simulink model "ADLK"  (R2022a)
settings: Solver=FixedStepDiscrete  StartTime=0.0  StopTime=10.0  FixedStep=0.01  RelTol=1e-3
libraries: simulink x4, DoorRatSts x4, ADLKDriver x2
settings Model: Creator=DELL  LastModifiedBy=DELL
settings DataIOCC: SaveFormat=StructureWithTime
settings OptimizationCC: DefaultParameterBehavior=Inlined  EnhancedBackFolding=on  PassReuseOutputArgsAs=Individual arguments  ZeroExternalMemoryAtStartup=off  ZeroInternalMemoryAtStartup=off  OptimizeBlockOrder=speed  DifferentSizesBufferReuse=on  OptimizationCustomize=off  EfficientTunableParamExpr=on
settings DebuggingCC: ParameterTunabilityLossMsg=error
settings ModelReferenceCC: ModelReferenceNumInstancesAllowed=Single
settings SFSimCC: MATLABDynamicMemAlloc=off
settings RTWCC: Description=AUTOSAR  SystemTargetFile=autosar.tlc  GenCodeOnly=on  TemplateMakefile=ert_default_tmf
settings CodeAppCC: ForceParamTrailComments=on  IgnoreCustomStorageClasses=off  OperatorAnnotations=on  SimulinkDataObjDesc=on  SFDataObjDesc=on  InsertBlockDesc=on
settings STFCustomTargetCC: TargetLangStandard=C99 (ISO)  MultiwordLength=256  ParMdlRefBuildCompliant=on  CompOptLevelCompliant=on  IncludeMdlTerminateFcn=off  CombineOutputUpdateFcns=on  SuppressErrorStatus=on  ERTCustomFileBanners=on  SupportNonFinite=off  SupportComplex=off  SupportContinuousTime=off  SupportNonInlinedSFcns=off  RemoveResetFunc=on  MATLABClassNameForMDSCustomization=Simulink.SoftwareTarget.ERTCustomization  AutosarCompliant=on  GRTInterface=off  UseToolchainInfoCompliant=on  LookupTableObjectStructAxisOrder=2,1,3,4,...  LUTObjectStructOrderEvenSpacing=Size,Table,Breakpoints  SystemTargetFile=autosar.tlc
settings ERTTargetCC: TargetLangStandard=C99 (ISO)  ConcurrentExecutionCompliant=off  IncludeMdlTerminateFcn=off  SuppressErrorStatus=on  SupportNonFinite=off  SupportComplex=off  ModelStepFunctionPrototypeControlCompliant=off  CPPClassGenCompliant=off  AutosarCompliant=on  LookupTableObjectStructAxisOrder=2,1,3,4,...  LUTObjectStructOrderEvenSpacing=Size,Table,Breakpoints  InlinedParameterPlacement=NonHierarchical  ERTCustomFileTemplate=example_file_process.tlc

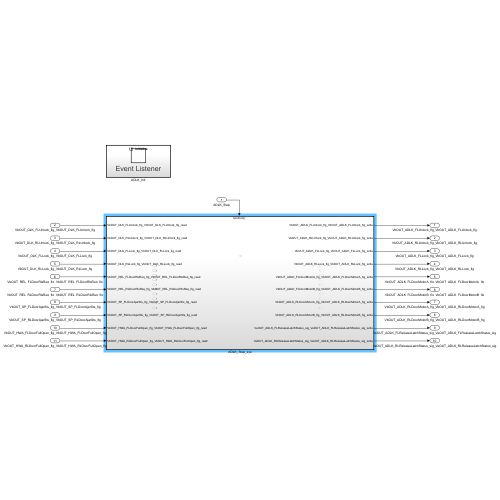
[thumbnail: Simulink's stored preview of the top-level diagram]
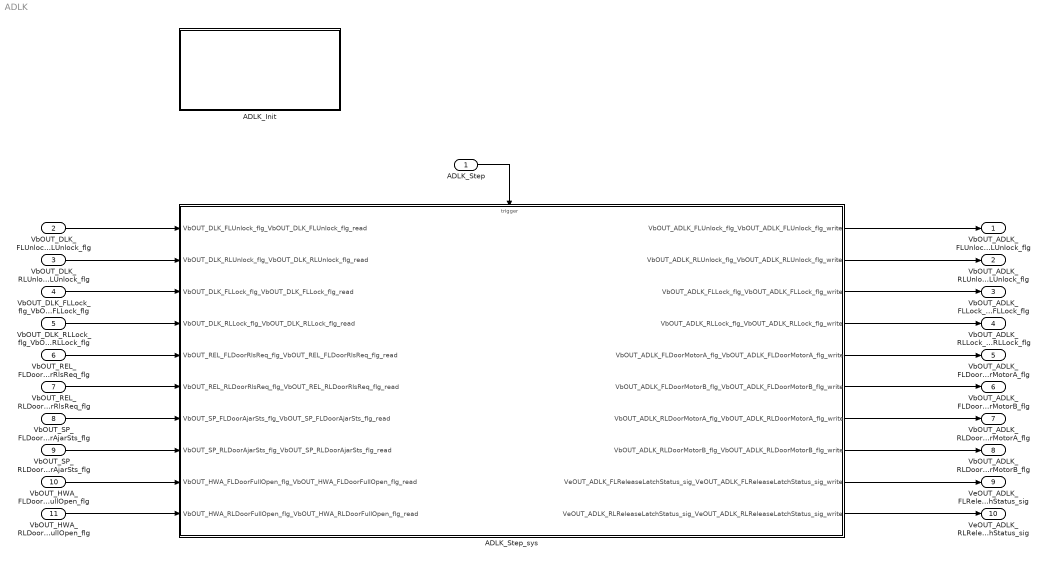
== system ADLK ==
  ADLK_Step : Inport  SampleTime=0.01  OutputFunctionCall=on
  VbOUT_DLK_FLUnlock_flg_VbOUT_DLK_FLUnlock_flg : Inport  Port=2  OutDataTypeStr=Boolean  PortDimensions=1
  VbOUT_DLK_RLUnlock_flg_VbOUT_DLK_RLUnlock_flg : Inport  Port=3  OutDataTypeStr=Boolean  PortDimensions=1
  VbOUT_DLK_FLLock_flg_VbOUT_DLK_FLLock_flg : Inport  Port=4  OutDataTypeStr=Boolean  PortDimensions=1
  VbOUT_DLK_RLLock_flg_VbOUT_DLK_RLLock_flg : Inport  Port=5  OutDataTypeStr=Boolean  PortDimensions=1
  VbOUT_REL_FLDoorRlsReq_flg_VbOUT_REL_FLDoorRlsReq_flg : Inport  Port=6  OutDataTypeStr=Boolean  PortDimensions=1
  VbOUT_REL_RLDoorRlsReq_flg_VbOUT_REL_RLDoorRlsReq_flg : Inport  Port=7  OutDataTypeStr=Boolean  PortDimensions=1
  VbOUT_SP_FLDoorAjarSts_flg_VbOUT_SP_FLDoorAjarSts_flg : Inport  Port=8  OutDataTypeStr=Boolean  PortDimensions=1
  VbOUT_SP_RLDoorAjarSts_flg_VbOUT_SP_RLDoorAjarSts_flg : Inport  Port=9  OutDataTypeStr=Boolean  PortDimensions=1
  VbOUT_HWA_FLDoorFullOpen_flg_VbOUT_HWA_FLDoorFullOpen_flg : Inport  Port=10  OutDataTypeStr=Boolean  PortDimensions=1
  VbOUT_HWA_RLDoorFullOpen_flg_VbOUT_HWA_RLDoorFullOpen_flg : Inport  Port=11  OutDataTypeStr=Boolean  PortDimensions=1
  ADLK_Init : Subsystem
  ADLK_Step_sys : Subsystem
  VbOUT_ADLK_FLUnlock_flg_VbOUT_ADLK_FLUnlock_flg : Outport  OutDataTypeStr=Boolean  PortDimensions=1
  VbOUT_ADLK_RLUnlock_flg_VbOUT_ADLK_RLUnlock_flg : Outport  Port=2  OutDataTypeStr=Boolean  PortDimensions=1
  VbOUT_ADLK_FLLock_flg_VbOUT_ADLK_FLLock_flg : Outport  Port=3  OutDataTypeStr=Boolean  PortDimensions=1
  VbOUT_ADLK_RLLock_flg_VbOUT_ADLK_RLLock_flg : Outport  Port=4  OutDataTypeStr=Boolean  PortDimensions=1
  VbOUT_ADLK_FLDoorMotorA_flg_VbOUT_ADLK_FLDoorMotorA_flg : Outport  Port=5  OutDataTypeStr=Boolean  PortDimensions=1
  VbOUT_ADLK_FLDoorMotorB_flg_VbOUT_ADLK_FLDoorMotorB_flg : Outport  Port=6  OutDataTypeStr=Boolean  PortDimensions=1
  VbOUT_ADLK_RLDoorMotorA_flg_VbOUT_ADLK_RLDoorMotorA_flg : Outport  Port=7  OutDataTypeStr=Boolean  PortDimensions=1
  VbOUT_ADLK_RLDoorMotorB_flg_VbOUT_ADLK_RLDoorMotorB_flg : Outport  Port=8  OutDataTypeStr=Boolean  PortDimensions=1
  VeOUT_ADLK_FLReleaseLatchStatus_sig_VeOUT_ADLK_FLReleaseLatchStatus_sig : Outport  Port=9  OutDataTypeStr=UInt8  PortDimensions=1
  VeOUT_ADLK_RLReleaseLatchStatus_sig_VeOUT_ADLK_RLReleaseLatchStatus_sig : Outport  Port=10  OutDataTypeStr=UInt8  PortDimensions=1
  wires:
  VbOUT_DLK_FLUnlock_flg_VbOUT_DLK_FLUnlock_flg/1 -> ADLK_Step_sys/1(VbOUT_DLK_FLUnlock_flg_VbOUT_DLK_FLUnlock_flg_read)
  VbOUT_DLK_RLUnlock_flg_VbOUT_DLK_RLUnlock_flg/1 -> ADLK_Step_sys/2(VbOUT_DLK_RLUnlock_flg_VbOUT_DLK_RLUnlock_flg_read)
  VbOUT_DLK_FLLock_flg_VbOUT_DLK_FLLock_flg/1 -> ADLK_Step_sys/3(VbOUT_DLK_FLLock_flg_VbOUT_DLK_FLLock_flg_read)
  VbOUT_DLK_RLLock_flg_VbOUT_DLK_RLLock_flg/1 -> ADLK_Step_sys/4(VbOUT_DLK_RLLock_flg_VbOUT_DLK_RLLock_flg_read)
  VbOUT_REL_FLDoorRlsReq_flg_VbOUT_REL_FLDoorRlsReq_flg/1 -> ADLK_Step_sys/5(VbOUT_REL_FLDoorRlsReq_flg_VbOUT_REL_FLDoorRlsReq_flg_read)
  VbOUT_REL_RLDoorRlsReq_flg_VbOUT_REL_RLDoorRlsReq_flg/1 -> ADLK_Step_sys/6(VbOUT_REL_RLDoorRlsReq_flg_VbOUT_REL_RLDoorRlsReq_flg_read)
  VbOUT_SP_FLDoorAjarSts_flg_VbOUT_SP_FLDoorAjarSts_flg/1 -> ADLK_Step_sys/7(VbOUT_SP_FLDoorAjarSts_flg_VbOUT_SP_FLDoorAjarSts_flg_read)
  VbOUT_SP_RLDoorAjarSts_flg_VbOUT_SP_RLDoorAjarSts_flg/1 -> ADLK_Step_sys/8(VbOUT_SP_RLDoorAjarSts_flg_VbOUT_SP_RLDoorAjarSts_flg_read)
  VbOUT_HWA_FLDoorFullOpen_flg_VbOUT_HWA_FLDoorFullOpen_flg/1 -> ADLK_Step_sys/9(VbOUT_HWA_FLDoorFullOpen_flg_VbOUT_HWA_FLDoorFullOpen_flg_read)
  VbOUT_HWA_RLDoorFullOpen_flg_VbOUT_HWA_RLDoorFullOpen_flg/1 -> ADLK_Step_sys/10(VbOUT_HWA_RLDoorFullOpen_flg_VbOUT_HWA_RLDoorFullOpen_flg_read)
  ADLK_Step_sys/1(VbOUT_ADLK_FLUnlock_flg_VbOUT_ADLK_FLUnlock_flg_write) -> VbOUT_ADLK_FLUnlock_flg_VbOUT_ADLK_FLUnlock_flg/1
  ADLK_Step_sys/2(VbOUT_ADLK_RLUnlock_flg_VbOUT_ADLK_RLUnlock_flg_write) -> VbOUT_ADLK_RLUnlock_flg_VbOUT_ADLK_RLUnlock_flg/1
  ADLK_Step_sys/3(VbOUT_ADLK_FLLock_flg_VbOUT_ADLK_FLLock_flg_write) -> VbOUT_ADLK_FLLock_flg_VbOUT_ADLK_FLLock_flg/1
  ADLK_Step_sys/4(VbOUT_ADLK_RLLock_flg_VbOUT_ADLK_RLLock_flg_write) -> VbOUT_ADLK_RLLock_flg_VbOUT_ADLK_RLLock_flg/1
  ADLK_Step_sys/5(VbOUT_ADLK_FLDoorMotorA_flg_VbOUT_ADLK_FLDoorMotorA_flg_write) -> VbOUT_ADLK_FLDoorMotorA_flg_VbOUT_ADLK_FLDoorMotorA_flg/1
  ADLK_Step_sys/6(VbOUT_ADLK_FLDoorMotorB_flg_VbOUT_ADLK_FLDoorMotorB_flg_write) -> VbOUT_ADLK_FLDoorMotorB_flg_VbOUT_ADLK_FLDoorMotorB_flg/1
  ADLK_Step_sys/7(VbOUT_ADLK_RLDoorMotorA_flg_VbOUT_ADLK_RLDoorMotorA_flg_write) -> VbOUT_ADLK_RLDoorMotorA_flg_VbOUT_ADLK_RLDoorMotorA_flg/1
  ADLK_Step_sys/8(VbOUT_ADLK_RLDoorMotorB_flg_VbOUT_ADLK_RLDoorMotorB_flg_write) -> VbOUT_ADLK_RLDoorMotorB_flg_VbOUT_ADLK_RLDoorMotorB_flg/1
  ADLK_Step_sys/9(VeOUT_ADLK_FLReleaseLatchStatus_sig_VeOUT_ADLK_FLReleaseLatchStatus_sig_write) -> VeOUT_ADLK_FLReleaseLatchStatus_sig_VeOUT_ADLK_FLReleaseLatchStatus_sig/1
  ADLK_Step_sys/10(VeOUT_ADLK_RLReleaseLatchStatus_sig_VeOUT_ADLK_RLReleaseLatchStatus_sig_write) -> VeOUT_ADLK_RLReleaseLatchStatus_sig_VeOUT_ADLK_RLReleaseLatchStatus_sig/1
  ADLK_Step/1 -> ADLK_Step_sys/Trigger

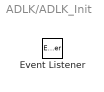
== system ADLK/ADLK_Init ==
  Event Listener : EventListener  EventName=reset

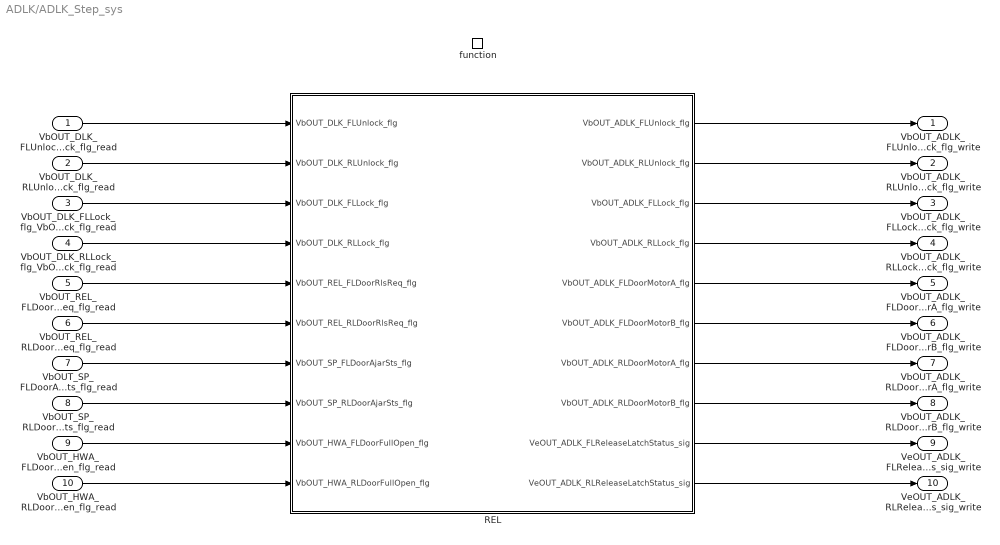
== system ADLK/ADLK_Step_sys ==
  VbOUT_DLK_FLUnlock_flg_VbOUT_DLK_FLUnlock_flg_read : Inport
  VbOUT_DLK_RLUnlock_flg_VbOUT_DLK_RLUnlock_flg_read : Inport  Port=2
  VbOUT_DLK_FLLock_flg_VbOUT_DLK_FLLock_flg_read : Inport  Port=3
  VbOUT_DLK_RLLock_flg_VbOUT_DLK_RLLock_flg_read : Inport  Port=4
  VbOUT_REL_FLDoorRlsReq_flg_VbOUT_REL_FLDoorRlsReq_flg_read : Inport  Port=5
  VbOUT_REL_RLDoorRlsReq_flg_VbOUT_REL_RLDoorRlsReq_flg_read : Inport  Port=6
  VbOUT_SP_FLDoorAjarSts_flg_VbOUT_SP_FLDoorAjarSts_flg_read : Inport  Port=7
  VbOUT_SP_RLDoorAjarSts_flg_VbOUT_SP_RLDoorAjarSts_flg_read : Inport  Port=8
  VbOUT_HWA_FLDoorFullOpen_flg_VbOUT_HWA_FLDoorFullOpen_flg_read : Inport  Port=9
  VbOUT_HWA_RLDoorFullOpen_flg_VbOUT_HWA_RLDoorFullOpen_flg_read : Inport  Port=10
  function : TriggerPort  TriggerType=function-call  VariantControl=(inherit)  SampleTimeType=periodic  SampleTime=-1
  REL : Subsystem
  VbOUT_ADLK_FLUnlock_flg_VbOUT_ADLK_FLUnlock_flg_write : Outport
      settings: EnsureOutportIsVirtual=on
  VbOUT_ADLK_RLUnlock_flg_VbOUT_ADLK_RLUnlock_flg_write : Outport  Port=2
      settings: EnsureOutportIsVirtual=on
  VbOUT_ADLK_FLLock_flg_VbOUT_ADLK_FLLock_flg_write : Outport  Port=3
      settings: EnsureOutportIsVirtual=on
  VbOUT_ADLK_RLLock_flg_VbOUT_ADLK_RLLock_flg_write : Outport  Port=4
      settings: EnsureOutportIsVirtual=on
  VbOUT_ADLK_FLDoorMotorA_flg_VbOUT_ADLK_FLDoorMotorA_flg_write : Outport  Port=5
      settings: EnsureOutportIsVirtual=on
  VbOUT_ADLK_FLDoorMotorB_flg_VbOUT_ADLK_FLDoorMotorB_flg_write : Outport  Port=6
      settings: EnsureOutportIsVirtual=on
  VbOUT_ADLK_RLDoorMotorA_flg_VbOUT_ADLK_RLDoorMotorA_flg_write : Outport  Port=7
      settings: EnsureOutportIsVirtual=on
  VbOUT_ADLK_RLDoorMotorB_flg_VbOUT_ADLK_RLDoorMotorB_flg_write : Outport  Port=8
      settings: EnsureOutportIsVirtual=on
  VeOUT_ADLK_FLReleaseLatchStatus_sig_VeOUT_ADLK_FLReleaseLatchStatus_sig_write : Outport  Port=9
      settings: EnsureOutportIsVirtual=on
  VeOUT_ADLK_RLReleaseLatchStatus_sig_VeOUT_ADLK_RLReleaseLatchStatus_sig_write : Outport  Port=10
      settings: EnsureOutportIsVirtual=on
  wires:
  REL/1(VbOUT_ADLK_FLUnlock_flg) -> VbOUT_ADLK_FLUnlock_flg_VbOUT_ADLK_FLUnlock_flg_write/1
  REL/2(VbOUT_ADLK_RLUnlock_flg) -> VbOUT_ADLK_RLUnlock_flg_VbOUT_ADLK_RLUnlock_flg_write/1
  REL/3(VbOUT_ADLK_FLLock_flg) -> VbOUT_ADLK_FLLock_flg_VbOUT_ADLK_FLLock_flg_write/1
  REL/4(VbOUT_ADLK_RLLock_flg) -> VbOUT_ADLK_RLLock_flg_VbOUT_ADLK_RLLock_flg_write/1
  REL/5(VbOUT_ADLK_FLDoorMotorA_flg) -> VbOUT_ADLK_FLDoorMotorA_flg_VbOUT_ADLK_FLDoorMotorA_flg_write/1
  REL/6(VbOUT_ADLK_FLDoorMotorB_flg) -> VbOUT_ADLK_FLDoorMotorB_flg_VbOUT_ADLK_FLDoorMotorB_flg_write/1
  REL/7(VbOUT_ADLK_RLDoorMotorA_flg) -> VbOUT_ADLK_RLDoorMotorA_flg_VbOUT_ADLK_RLDoorMotorA_flg_write/1
  REL/8(VbOUT_ADLK_RLDoorMotorB_flg) -> VbOUT_ADLK_RLDoorMotorB_flg_VbOUT_ADLK_RLDoorMotorB_flg_write/1
  REL/9(VeOUT_ADLK_FLReleaseLatchStatus_sig) -> VeOUT_ADLK_FLReleaseLatchStatus_sig_VeOUT_ADLK_FLReleaseLatchStatus_sig_write/1
  REL/10(VeOUT_ADLK_RLReleaseLatchStatus_sig) -> VeOUT_ADLK_RLReleaseLatchStatus_sig_VeOUT_ADLK_RLReleaseLatchStatus_sig_write/1
  VbOUT_DLK_FLUnlock_flg_VbOUT_DLK_FLUnlock_flg_read/1 -> REL/1(VbOUT_DLK_FLUnlock_flg)
  VbOUT_DLK_RLUnlock_flg_VbOUT_DLK_RLUnlock_flg_read/1 -> REL/2(VbOUT_DLK_RLUnlock_flg)
  VbOUT_DLK_FLLock_flg_VbOUT_DLK_FLLock_flg_read/1 -> REL/3(VbOUT_DLK_FLLock_flg)
  VbOUT_DLK_RLLock_flg_VbOUT_DLK_RLLock_flg_read/1 -> REL/4(VbOUT_DLK_RLLock_flg)
  VbOUT_REL_FLDoorRlsReq_flg_VbOUT_REL_FLDoorRlsReq_flg_read/1 -> REL/5(VbOUT_REL_FLDoorRlsReq_flg)
  VbOUT_REL_RLDoorRlsReq_flg_VbOUT_REL_RLDoorRlsReq_flg_read/1 -> REL/6(VbOUT_REL_RLDoorRlsReq_flg)
  VbOUT_SP_FLDoorAjarSts_flg_VbOUT_SP_FLDoorAjarSts_flg_read/1 -> REL/7(VbOUT_SP_FLDoorAjarSts_flg)
  VbOUT_SP_RLDoorAjarSts_flg_VbOUT_SP_RLDoorAjarSts_flg_read/1 -> REL/8(VbOUT_SP_RLDoorAjarSts_flg)
  VbOUT_HWA_FLDoorFullOpen_flg_VbOUT_HWA_FLDoorFullOpen_flg_read/1 -> REL/9(VbOUT_HWA_FLDoorFullOpen_flg)
  VbOUT_HWA_RLDoorFullOpen_flg_VbOUT_HWA_RLDoorFullOpen_flg_read/1 -> REL/10(VbOUT_HWA_RLDoorFullOpen_flg)

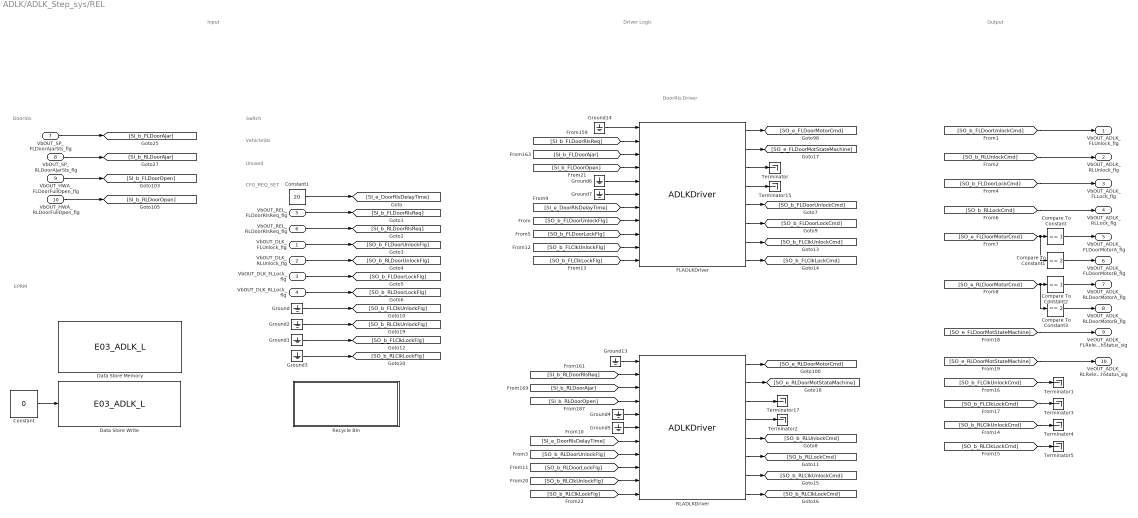
== system ADLK/ADLK_Step_sys/REL ==
  note: VehicleSts
  note: Input
  note: Output
  note: EPRM
  note: Driver Logic
  note: DoorRls Driver
  note: Switch
  note: DoorSts
  note: CFG_REQ_SET
  note: Unused
  VbOUT_DLK_FLUnlock_flg : Inport
  VbOUT_DLK_RLUnlock_flg : Inport  Port=2
  VbOUT_DLK_FLLock_flg : Inport  Port=3
  VbOUT_DLK_RLLock_flg : Inport  Port=4
  VbOUT_REL_FLDoorRlsReq_flg : Inport  Port=5
  VbOUT_REL_RLDoorRlsReq_flg : Inport  Port=6
  VbOUT_SP_FLDoorAjarSts_flg : Inport  Port=7
  VbOUT_SP_RLDoorAjarSts_flg : Inport  Port=8
  VbOUT_HWA_FLDoorFullOpen_flg : Inport  Port=9
  VbOUT_HWA_RLDoorFullOpen_flg : Inport  Port=10
  Compare To Constant : simulink/Logic and Bit Operations/Compare To Constant  relop===  const=1  OutDataTypeStr=boolean
  Compare To Constant1 : simulink/Logic and Bit Operations/Compare To Constant  relop===  const=2  OutDataTypeStr=boolean
  Compare To Constant2 : simulink/Logic and Bit Operations/Compare To Constant  relop===  const=1  OutDataTypeStr=boolean
  Compare To Constant3 : simulink/Logic and Bit Operations/Compare To Constant  relop===  const=2  OutDataTypeStr=boolean
  Constant : Constant  Value=0  OutDataTypeStr=uint8
  Constant1 : Constant  Value=20  OutDataTypeStr=uint8
  Data Store Memory : DataStoreMemory  DataStoreName=E03_ADLK_L  WriteAfterWriteMsg=warning  ShowAdditionalParam=off  OutDataTypeStr=uint8
  Data Store Write : DataStoreWrite  DataStoreName=E03_ADLK_L  IndexOptions=Index vector (dialog)  Indices=1  OutputSizes=1
  FLADLKDriver : ADLKDriver/ADLKDriver  SystemSampleTime=-1  VariantActivationTime=update diagram  Latency=0  AutoFrameSizeCalculation=off
  Ground{,1..7,13..14} (10 alike) : Ground
  RLADLKDriver : ADLKDriver/ADLKDriver  SystemSampleTime=-1  VariantActivationTime=update diagram  Latency=0  AutoFrameSizeCalculation=off
  Recycle Bin : Subsystem
  Terminator{,1..5,15,17} (8 alike) : Terminator
  VbOUT_ADLK_FLUnlock_flg : Outport
  VbOUT_ADLK_RLUnlock_flg : Outport  Port=2
  VbOUT_ADLK_FLLock_flg : Outport  Port=3
  VbOUT_ADLK_RLLock_flg : Outport  Port=4
  VbOUT_ADLK_FLDoorMotorA_flg : Outport  Port=5
  VbOUT_ADLK_FLDoorMotorB_flg : Outport  Port=6
  VbOUT_ADLK_RLDoorMotorA_flg : Outport  Port=7
  VbOUT_ADLK_RLDoorMotorB_flg : Outport  Port=8
  VeOUT_ADLK_FLReleaseLatchStatus_sig : Outport  Port=9
  VeOUT_ADLK_RLReleaseLatchStatus_sig : Outport  Port=10
  wires:
  Constant/1 -> Data Store Write/1
  [SI_b_RLDoorOpen] -> RLADLKDriver/4
  [SI_b_RLDoorAjar] -> RLADLKDriver/3
  [SI_b_RLDoorRlsReq] -> RLADLKDriver/2
  Ground13/1 -> RLADLKDriver/1
  [SI_b_FLDoorAjar] -> FLADLKDriver/3
  [SI_b_FLDoorRlsReq] -> FLADLKDriver/2
  [SI_b_FLDoorOpen] -> FLADLKDriver/4
  [SI_e_DoorRlsDelayTime] -> FLADLKDriver/7
  Ground4/1 -> RLADLKDriver/5
  Ground5/1 -> RLADLKDriver/6
  Ground6/1 -> FLADLKDriver/5
  Ground7/1 -> FLADLKDriver/6
  Ground14/1 -> FLADLKDriver/1
  Constant1/1 -> [SI_e_DoorRlsDelayTime]
  [SI_e_DoorRlsDelayTime] -> RLADLKDriver/7
  VbOUT_SP_FLDoorAjarSts_flg/1 -> [SI_b_FLDoorAjar]
  VbOUT_SP_RLDoorAjarSts_flg/1 -> [SI_b_RLDoorAjar]
  VbOUT_HWA_FLDoorFullOpen_flg/1 -> [SI_b_FLDoorOpen]
  VbOUT_HWA_RLDoorFullOpen_flg/1 -> [SI_b_RLDoorOpen]
  VbOUT_REL_FLDoorRlsReq_flg/1 -> [SI_b_FLDoorRlsReq]
  VbOUT_REL_RLDoorRlsReq_flg/1 -> [SI_b_RLDoorRlsReq]
  [SO_b_FLDoorLockFlg] -> FLADLKDriver/9
  [SO_b_FLDoorUnlockFlg] -> FLADLKDriver/8
  [SO_b_RLDoorUnlockFlg] -> RLADLKDriver/8
  [SO_b_RLDoorLockFlg] -> RLADLKDriver/9
  VbOUT_DLK_FLUnlock_flg/1 -> [SO_b_FLDoorUnlockFlg]
  VbOUT_DLK_RLUnlock_flg/1 -> [SO_b_RLDoorUnlockFlg]
  VbOUT_DLK_FLLock_flg/1 -> [SO_b_FLDoorLockFlg]
  VbOUT_DLK_RLLock_flg/1 -> [SO_b_RLDoorLockFlg]
  [SO_b_FLClkUnlockFlg] -> FLADLKDriver/10
  [SO_b_FLClkLockFlg] -> FLADLKDriver/11
  Ground/1 -> [SO_b_FLClkUnlockFlg]
  Ground1/1 -> [SO_b_FLClkLockFlg]
  [SO_b_FLDoorUnlockCmd] -> VbOUT_ADLK_FLUnlock_flg/1
  [SO_b_RLUnlockCmd] -> VbOUT_ADLK_RLUnlock_flg/1
  [SO_b_FLDoorLockCmd] -> VbOUT_ADLK_FLLock_flg/1
  [SO_b_RLLockCmd] -> VbOUT_ADLK_RLLock_flg/1
  [SO_e_FLDoorMotorCmd] -> Compare To Constant1/1, Compare To Constant/1
  Compare To Constant/1 -> VbOUT_ADLK_FLDoorMotorA_flg/1
  Compare To Constant1/1 -> VbOUT_ADLK_FLDoorMotorB_flg/1
  Compare To Constant2/1 -> VbOUT_ADLK_RLDoorMotorA_flg/1
  [SO_e_RLDoorMotorCmd] -> Compare To Constant3/1, Compare To Constant2/1
  Compare To Constant3/1 -> VbOUT_ADLK_RLDoorMotorB_flg/1
  [SO_e_FLDoorMotStateMachine] -> VeOUT_ADLK_FLReleaseLatchStatus_sig/1
  [SO_e_RLDoorMotStateMachine] -> VeOUT_ADLK_RLReleaseLatchStatus_sig/1
  [SO_b_FLClkUnlockCmd] -> Terminator1/1
  [SO_b_FLClkLockCmd] -> Terminator3/1
  [SO_b_RLClkUnlockCmd] -> Terminator4/1
  [SO_b_RLClkLockCmd] -> Terminator5/1
  FLADLKDriver/1 -> [SO_e_FLDoorMotorCmd]
  FLADLKDriver/8 -> [SO_b_FLClkLockCmd]
  FLADLKDriver/7 -> [SO_b_FLClkUnlockCmd]
  FLADLKDriver/2 -> [SO_e_FLDoorMotStateMachine]
  FLADLKDriver/6 -> [SO_b_FLDoorLockCmd]
  FLADLKDriver/5 -> [SO_b_FLDoorUnlockCmd]
  FLADLKDriver/4 -> Terminator15/1
  FLADLKDriver/3 -> Terminator/1
  RLADLKDriver/1 -> [SO_e_RLDoorMotorCmd]
  RLADLKDriver/8 -> [SO_b_RLClkLockCmd]
  RLADLKDriver/7 -> [SO_b_RLClkUnlockCmd]
  RLADLKDriver/6 -> [SO_b_RLLockCmd]
  RLADLKDriver/2 -> [SO_e_RLDoorMotStateMachine]
  RLADLKDriver/5 -> [SO_b_RLUnlockCmd]
  RLADLKDriver/4 -> Terminator2/1
  RLADLKDriver/3 -> Terminator17/1
  Ground2/1 -> [SO_b_RLClkUnlockFlg]
  Ground3/1 -> [SO_b_RLClkLockFlg]
  [SO_b_RLClkUnlockFlg] -> RLADLKDriver/10
  [SO_b_RLClkLockFlg] -> RLADLKDriver/11

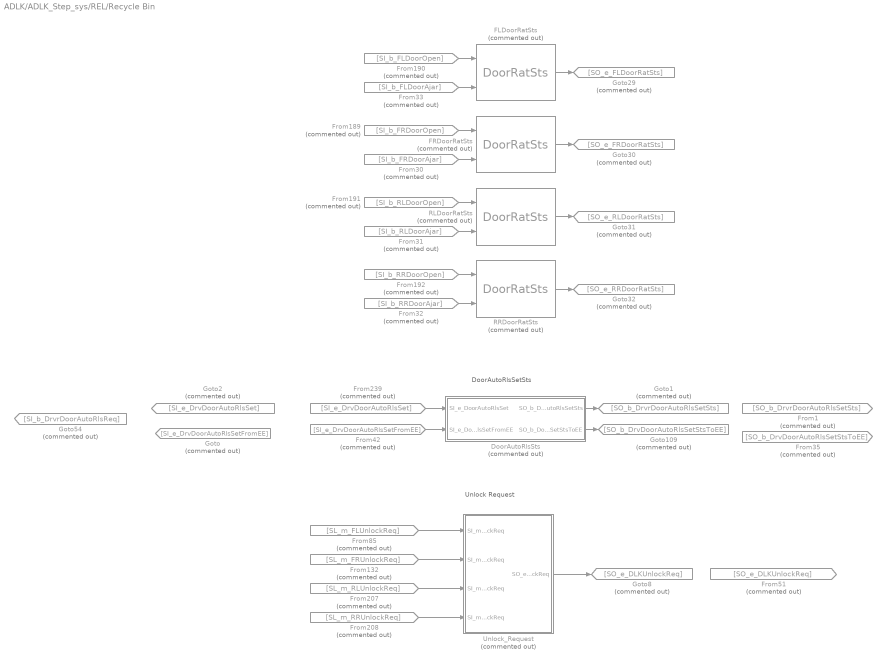
== system ADLK/ADLK_Step_sys/REL/Recycle Bin ==
  note: DoorAutoRlsSetSts
  note: Unlock Request
  DoorAutoRlsSts : Stateflow chart  Commented=on  TreatAsAtomicUnit=on
  FLDoorRatSts : DoorRatSts/DoorRatSts  Commented=on  SystemSampleTime=-1  VariantActivationTime=update diagram  Latency=0  AutoFrameSizeCalculation=off
  FRDoorRatSts : DoorRatSts/DoorRatSts  Commented=on  SystemSampleTime=-1  VariantActivationTime=update diagram  Latency=0  AutoFrameSizeCalculation=off
  From1 : From  Commented=on  GotoTag=SO_b_DrvrDoorAutoRlsSetSts
  From132 : From  Commented=on  GotoTag=SL_m_FRUnlockReq
  From189 : From  Commented=on  GotoTag=SI_b_FRDoorOpen
  From190 : From  Commented=on  GotoTag=SI_b_FLDoorOpen
  From191 : From  Commented=on  GotoTag=SI_b_RLDoorOpen
  From192 : From  Commented=on  GotoTag=SI_b_RRDoorOpen
  From207 : From  Commented=on  GotoTag=SL_m_RLUnlockReq
  From208 : From  Commented=on  GotoTag=SL_m_RRUnlockReq
  From239 : From  Commented=on  GotoTag=SI_e_DrvDoorAutoRlsSet
  From30 : From  Commented=on  GotoTag=SI_b_FRDoorAjar
  From31 : From  Commented=on  GotoTag=SI_b_RLDoorAjar
  From32 : From  Commented=on  GotoTag=SI_b_RRDoorAjar
  From33 : From  Commented=on  GotoTag=SI_b_FLDoorAjar
  From35 : From  Commented=on  GotoTag=SO_b_DrvDoorAutoRlsSetStsToEE
  From42 : From  Commented=on  GotoTag=SI_e_DrvDoorAutoRlsSetFromEE
  From51 : From  Commented=on  GotoTag=SO_e_DLKUnlockReq
  From85 : From  Commented=on  GotoTag=SL_m_FLUnlockReq
  Goto : Goto  Commented=on  GotoTag=SI_e_DrvDoorAutoRlsSetFromEE
  Goto1 : Goto  Commented=on  GotoTag=SO_b_DrvrDoorAutoRlsSetSts
  Goto109 : Goto  Commented=on  GotoTag=SO_b_DrvDoorAutoRlsSetStsToEE
  Goto2 : Goto  Commented=on  GotoTag=SI_e_DrvDoorAutoRlsSet
  Goto29 : Goto  Commented=on  GotoTag=SO_e_FLDoorRatSts
  Goto30 : Goto  Commented=on  GotoTag=SO_e_FRDoorRatSts
  Goto31 : Goto  Commented=on  GotoTag=SO_e_RLDoorRatSts
  Goto32 : Goto  Commented=on  GotoTag=SO_e_RRDoorRatSts
  Goto54 : Goto  Commented=on  GotoTag=SI_b_DrvrDoorAutoRlsReq
  Goto8 : Goto  Commented=on  GotoTag=SO_e_DLKUnlockReq
  RLDoorRatSts : DoorRatSts/DoorRatSts  Commented=on  SystemSampleTime=-1  VariantActivationTime=update diagram  Latency=0  AutoFrameSizeCalculation=off
  RRDoorRatSts : DoorRatSts/DoorRatSts  Commented=on  SystemSampleTime=-1  VariantActivationTime=update diagram  Latency=0  AutoFrameSizeCalculation=off
  Unlock_Request : Stateflow chart  Commented=on  TreatAsAtomicUnit=on
  wires:
  FLDoorRatSts/1 -> Goto29/1
  From191/1 -> RLDoorRatSts/1
  FRDoorRatSts/1 -> Goto30/1
  From190/1 -> FLDoorRatSts/1
  From192/1 -> RRDoorRatSts/1
  From189/1 -> FRDoorRatSts/1
  RRDoorRatSts/1 -> Goto32/1
  RLDoorRatSts/1 -> Goto31/1
  From30/1 -> FRDoorRatSts/2
  From32/1 -> RRDoorRatSts/2
  From31/1 -> RLDoorRatSts/2
  From33/1 -> FLDoorRatSts/2
  DoorAutoRlsSts/1(SO_b_DoorAutoRlsSetSts) -> Goto1/1
  DoorAutoRlsSts/2(SO_b_DoorAutoRlsSetStsToEE) -> Goto109/1
  From42/1 -> DoorAutoRlsSts/2(SI_e_DoorAutoRlsSetFromEE)
  From239/1 -> DoorAutoRlsSts/1(SI_e_DoorAutoRlsSet)
  From132/1 -> Unlock_Request/2(SI_m_FRUnlockReq)
  From208/1 -> Unlock_Request/4(SI_m_RRUnlockReq)
  From207/1 -> Unlock_Request/3(SI_m_RLUnlockReq)
  Unlock_Request/1(SO_e_UnlockReq) -> Goto8/1
  From85/1 -> Unlock_Request/1(SI_m_FLUnlockReq)

== stateflow chart ADLK/ADLK_Step_sys/REL/Recycle Bin/DoorAutoRlsSts ==
  state DoorLockSet
    (default) -> (junction 127) : /* DoorLockSet */
    DoorLockSet -> (junction 127)
    (junction 127) -> (junction 128) [order 1] : [SI_e_DoorAutoRlsSet == 1 || ...
        | (SI_e_DoorAutoRlsSet != 2 && SL_e_DoorAutoRlsSetBackup == 1)]
    (junction 127) -> (junction 129) [order 2]
    (junction 128) -> (junction 136) : {SO_b_DoorAutoRlsSetSts = 1; ...
        | SO_b_DoorAutoRlsSetStsToEE = 1; ...
        | SL_e_DoorAutoRlsSetBackup = 1}
    (junction 129) -> (junction 130) [order 1] : [SI_e_DoorAutoRlsSet == 2 || ...
        | (SI_e_DoorAutoRlsSet != 1 && SL_e_DoorAutoRlsSetBackup == 2)]
    (junction 129) -> (junction 131) [order 2]
    (junction 130) -> (junction 135) : {SO_b_DoorAutoRlsSetSts = 0; ...
        | SO_b_DoorAutoRlsSetStsToEE = 0; ...
        | SL_e_DoorAutoRlsSetBackup = 2}
    (junction 131) -> (junction 132) [order 1] : [SI_e_DoorAutoRlsSetFromEE == 1]
    (junction 131) -> (junction 151) [order 2]
    (junction 132) -> (junction 134) : {SO_b_DoorAutoRlsSetSts = 1; ...
        | SO_b_DoorAutoRlsSetStsToEE = 1;}
    (junction 151) -> (junction 159) [order 1] : [SI_e_DoorAutoRlsSetFromEE == 0]
    (junction 151) -> (junction 133) [order 2]
    (junction 159) -> (junction 160) : {SO_b_DoorAutoRlsSetSts = 0; ...
        | SO_b_DoorAutoRlsSetStsToEE = 0;}
    (junction 160) -> (junction 133)
    (junction 134) -> (junction 160)
    (junction 135) -> (junction 134)
    (junction 136) -> (junction 135)
    (junction 133) -> (junction 137)
  data: SO_b_DoorAutoRlsSetSts output boolean; SI_e_DoorAutoRlsSet input uint8; SI_e_DoorAutoRlsSetFromEE input uint8; SO_b_DoorAutoRlsSetStsToEE output boolean; SL_e_DoorAutoRlsSetBackup local uint8 =0

== stateflow chart ADLK/ADLK_Step_sys/REL/Recycle Bin/Unlock_Request ==
  state req = GetDrvUnlockReq [function]
    (default) -> (junction 216)
    (junction 216) -> (junction 217) [order 1] : [SI_m_FLUnlockReq == Unlock_PE]
    (junction 216) -> (junction 218) [order 2]
    (junction 217) -> (junction 222) : {req = Unlock_PE;}
    (junction 218) -> (junction 219) [order 1] : [SI_m_FLUnlockReq == Unlock_Req]
    (junction 218) -> (junction 220) [order 2] : {req = Unlock_Idle;}
    (junction 219) -> (junction 221) : {req = Unlock_Req;}
    (junction 221) -> (junction 220)
    (junction 222) -> (junction 221)
    (junction 220) -> (junction 223)
  state UnlockReq
    (default) -> (junction 185)
    UnlockReq -> (junction 185)
    (junction 185) -> (junction 186) [order 1] : [(GetDrvUnlockReq() == Unlock_Req && GetPassUnlockReq() == Unlock_Req) || ...
        | GetDrvUnlockReq() == Unlock_PE || ...
        | GetPassUnlockReq() == Unlock_PE]
    (junction 185) -> (junction 187) [order 2]
    (junction 186) -> (junction 194) : {SO_e_UnlockReq = 3;}
    (junction 187) -> (junction 188) [order 1] : [GetDrvUnlockReq() == Unlock_Idle && ...
        | GetPassUnlockReq() == Unlock_Req]
    (junction 187) -> (junction 189) [order 2]
    (junction 188) -> (junction 193) : {SO_e_UnlockReq = 2;}
    (junction 189) -> (junction 190) [order 1] : [GetDrvUnlockReq() == Unlock_Req && ...
        | GetPassUnlockReq() == Unlock_Idle]
    (junction 189) -> (junction 191) [order 2] : {SO_e_UnlockReq = 0;}
    (junction 190) -> (junction 192) : {SO_e_UnlockReq = 1;}
    (junction 192) -> (junction 191)
    (junction 193) -> (junction 192)
    (junction 194) -> (junction 193)
    (junction 191) -> (junction 195)
  state req = GetPassUnlockReq [function]
    (default) -> (junction 232)
    (junction 232) -> (junction 228) [order 1] : [SI_m_FRUnlockReq == Unlock_PE || ...
        | SI_m_RLUnlockReq == Unlock_PE || ...
        | SI_m_RRUnlockReq == Unlock_PE]
    (junction 232) -> (junction 234) [order 2]
    (junction 228) -> (junction 238) : {req = Unlock_PE;}
    (junction 234) -> (junction 237) [order 1] : [SI_m_FRUnlockReq == Unlock_Req || ...
        | SI_m_RLUnlockReq == Unlock_Req || ...
        | SI_m_RRUnlockReq == Unlock_Req]
    (junction 234) -> (junction 240) [order 2] : {req = Unlock_Idle;}
    (junction 237) -> (junction 241) : {req = Unlock_Req;}
    (junction 241) -> (junction 240)
    (junction 238) -> (junction 241)
    (junction 240) -> (junction 239)
  data: req function_output double; req function_output double; SO_e_UnlockReq output uint8; SI_m_FLUnlockReq input Enum: Unlock_Req_E; SI_m_FRUnlockReq input Enum: Unlock_Req_E; SI_m_RLUnlockReq input Enum: Unlock_Req_E; SI_m_RRUnlockReq input Enum: Unlock_Req_E
